simulink model "ieee80211n"  (Simulink 6.0)
settings: Solver=VariableStepDiscrete  StartTime=0.0  StopTime=inf  RelTol=1e-3
PreLoadFcn:
  | load IEEE80211n_init;
values from neighbouring files (symbols this model uses):
  params =     [IEEE80211n_init.mat]    (also in IEEE80211n_settings.m = p)
undefined symbols (not defined in the file or in its folder): magnitude
libraries: commblkintrlv2 x196, dspsigops x143, simulink x136, commdigbbndam2 x98, dspmtrx3 x96, dspsigattribs x69, dspstat3 x38, commutil2 x32, commsequence2 x26, commcnvcod2 x10, dspindex x9, dspmlti3 x8
(part 3 of 12)

== system ieee80211n/cyclic prefix1 ==
  in : Inport  Port=1  LatchInput=off
  Add Cyclic Prefix : Selector  InputType=Matrix  Elements=[49:64 1:64]  Rows=params.TXCyclicPrefixIndices  Columns=-1  InputPortWidth=64
  "Cyclic shift, SS2" : Subsystem
      mask Display: disp('Cyclic Shift\nDelay')
  out : Outport
  wires:
  Add Cyclic Prefix/1 -> out/1
  in/1 -> "Cyclic shift, SS2"/1(in)
  "Cyclic shift, SS2"/1(out) -> Add Cyclic Prefix/1

== system ieee80211n/cyclic prefix2 ==
  in : Inport  Port=1  LatchInput=off
  Add Cyclic Prefix : Selector  InputType=Matrix  Elements=[49:64 1:64]  Rows=params.TXCyclicPrefixIndices  Columns=-1  InputPortWidth=64
  "Cyclic shift, SS3" : Subsystem
      mask Display: disp('Cyclic Shift\nDelay')
  out : Outport
  wires:
  Add Cyclic Prefix/1 -> out/1
  in/1 -> "Cyclic shift, SS3"/1(in)
  "Cyclic shift, SS3"/1(out) -> Add Cyclic Prefix/1

== system ieee80211n/cyclic prefix3 ==
  in : Inport  Port=1  LatchInput=off
  Add Cyclic Prefix : Selector  InputType=Matrix  Elements=[49:64 1:64]  Rows=params.TXCyclicPrefixIndices  Columns=-1  InputPortWidth=64
  "Cyclic shift, SS4" : Subsystem
      mask Display: disp('Cyclic Shift\nDelay')
  out : Outport
  wires:
  Add Cyclic Prefix/1 -> out/1
  in/1 -> "Cyclic shift, SS4"/1(in)
  "Cyclic shift, SS4"/1(out) -> Add Cyclic Prefix/1

== system ieee80211n/remove cyclic prefix ==
  In1 : Inport  Port=1  LatchInput=off
  Remove cyclic prefix : Selector  InputType=Matrix  Elements=[17:80]  Rows=params.RXCyclicPrefixIndices  Columns=-1  InputPortWidth=80
  Out1 : Outport
  wires:
  In1/1 -> Remove cyclic prefix/1
  Remove cyclic prefix/1 -> Out1/1

== system ieee80211n/remove cyclic prefix1 ==
  In1 : Inport  Port=1  LatchInput=off
  Remove cyclic prefix : Selector  InputType=Matrix  Elements=[17:80]  Rows=params.RXCyclicPrefixIndices  Columns=-1  InputPortWidth=80
  Out1 : Outport
  wires:
  In1/1 -> Remove cyclic prefix/1
  Remove cyclic prefix/1 -> Out1/1

== system ieee80211n/remove cyclic prefix2 ==
  In1 : Inport  Port=1  LatchInput=off
  Remove cyclic prefix : Selector  InputType=Matrix  Elements=[17:80]  Rows=params.RXCyclicPrefixIndices  Columns=-1  InputPortWidth=80
  Out1 : Outport
  wires:
  In1/1 -> Remove cyclic prefix/1
  Remove cyclic prefix/1 -> Out1/1

== system ieee80211n/remove cyclic prefix3 ==
  In1 : Inport  Port=1  LatchInput=off
  Remove cyclic prefix : Selector  InputType=Matrix  Elements=[17:80]  Rows=params.RXCyclicPrefixIndices  Columns=-1  InputPortWidth=80
  Out1 : Outport
  wires:
  In1/1 -> Remove cyclic prefix/1
  Remove cyclic prefix/1 -> Out1/1

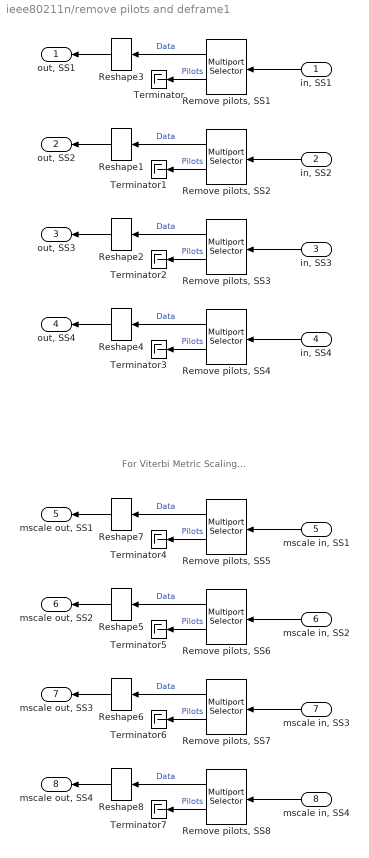
== system ieee80211n/remove pilots and deframe1 ==
  note: For Viterbi Metric Scaling...
  "in, SS1" : Inport  Orientation=left  Port=1  LatchInput=off
  "in, SS2" : Inport  Orientation=left  Port=2  LatchInput=off
  "in, SS3" : Inport  Orientation=left  Port=3  LatchInput=off
  "in, SS4" : Inport  Orientation=left  Port=4  LatchInput=off
  "mscale in, SS1" : Inport  Orientation=left  Port=5  LatchInput=off
  "mscale in, SS2" : Inport  Orientation=left  Port=6  LatchInput=off
  "mscale in, SS3" : Inport  Orientation=left  Port=7  LatchInput=off
  "mscale in, SS4" : Inport  Orientation=left  Port=8  LatchInput=off
  Remove pilots, SS{1..8} (8 alike) : dspindex/Multiport Selector  Orientation=left  rowsOrCols=Rows  idxCellArray="{[1:7 9:21 23:34 36:48 50:56], [8 22 35 49]}  % {[1:5 7:19 21:32 34:46 48:52], [6 20 33 47]}"  idxErrMode=Clip Index
  Reshape{1..8} (8 alike) : simulink/Math Operations/Reshape  Orientation=left  OutputDimensionality=Column vector  OutputDimensions=960
  Terminator{,1..7} (8 alike) : Terminator
  "out, SS1" : Outport  Orientation=left
  "out, SS2" : Outport  Orientation=left  Port=2
  "out, SS3" : Outport  Orientation=left  Port=3
  "out, SS4" : Outport  Orientation=left  Port=4
  "mscale out, SS1" : Outport  Orientation=left  Port=5
  "mscale out, SS2" : Outport  Orientation=left  Port=6
  "mscale out, SS3" : Outport  Orientation=left  Port=7
  "mscale out, SS4" : Outport  Orientation=left  Port=8
  wires:
  "Remove pilots, SS1"/2 -> Terminator/1  "Pilots"
  "Remove pilots, SS1"/1 -> Reshape3/1  "Data"
  Reshape3/1 -> "out, SS1"/1
  "in, SS1"/1 -> "Remove pilots, SS1"/1
  "Remove pilots, SS2"/2 -> Terminator1/1  "Pilots"
  "Remove pilots, SS2"/1 -> Reshape1/1  "Data"
  Reshape1/1 -> "out, SS2"/1
  "in, SS2"/1 -> "Remove pilots, SS2"/1
  "Remove pilots, SS3"/2 -> Terminator2/1  "Pilots"
  "Remove pilots, SS3"/1 -> Reshape2/1  "Data"
  Reshape2/1 -> "out, SS3"/1
  "in, SS3"/1 -> "Remove pilots, SS3"/1
  "Remove pilots, SS4"/2 -> Terminator3/1  "Pilots"
  "Remove pilots, SS4"/1 -> Reshape4/1  "Data"
  Reshape4/1 -> "out, SS4"/1
  "in, SS4"/1 -> "Remove pilots, SS4"/1
  "Remove pilots, SS5"/2 -> Terminator4/1  "Pilots"
  "Remove pilots, SS5"/1 -> Reshape7/1  "Data"
  Reshape7/1 -> "mscale out, SS1"/1
  "mscale in, SS1"/1 -> "Remove pilots, SS5"/1
  "Remove pilots, SS6"/2 -> Terminator5/1  "Pilots"
  "Remove pilots, SS6"/1 -> Reshape5/1  "Data"
  Reshape5/1 -> "mscale out, SS2"/1
  "mscale in, SS2"/1 -> "Remove pilots, SS6"/1
  "Remove pilots, SS7"/2 -> Terminator6/1  "Pilots"
  "Remove pilots, SS7"/1 -> Reshape6/1  "Data"
  Reshape6/1 -> "mscale out, SS3"/1
  "mscale in, SS3"/1 -> "Remove pilots, SS7"/1
  "Remove pilots, SS8"/2 -> Terminator7/1  "Pilots"
  "Remove pilots, SS8"/1 -> Reshape8/1  "Data"
  Reshape8/1 -> "mscale out, SS4"/1
  "mscale in, SS4"/1 -> "Remove pilots, SS8"/1

== system ieee80211n/remove pilots and training ==
  in : Inport  Port=1  LatchInput=off
  Frame Status Conversion1 : dspsigattribs/Frame Status Conversion  growRefPort=off  outframe=Sample-based
  Remove DC component : Selector  InputType=Matrix  Elements=[1:26 27:]  Rows=[1:26 28:53]  Columns=-1  InputPortWidth=53
  Remove training and pilots : Selector  InputType=Matrix  Elements=[17:80]  Rows=[1:5 7:19 21:32 34:46 48:52]  Columns=params.OFDMTrainPerFrame+1:params.OFDMTotSymPerFrame  InputPortWidth=80
  Reshape5 : simulink/Math Operations/Reshape  OutputDimensionality=Column vector  OutputDimensions=960
  out : Outport
  wires:
  Remove training and pilots/1 -> Reshape5/1
  Remove DC component/1 -> Remove training and pilots/1
  in/1 -> Remove DC component/1
  Reshape5/1 -> Frame Status Conversion1/1
  Frame Status Conversion1/1 -> out/1

== system ieee80211n/training ==
  Frame Status Conversion{1..4} (4 alike) : dspsigattribs/Frame Status Conversion  Orientation=left  growRefPort=off  outframe=Frame-based
  "Training, SS1" : Constant  Orientation=left  Value=params.HT20_long_training_seq_ss1
  "Training, SS2" : Constant  Orientation=left  Value=params.HT20_long_training_seq_ss2
  "Training, SS3" : Constant  Orientation=left  Value=params.HT20_long_training_seq_ss3
  "Training, SS4" : Constant  Orientation=left  Value=params.HT20_long_training_seq_ss4
  "Out, SS1" : Outport  Orientation=left
  "Out, SS2" : Outport  Orientation=left  Port=2
  "Out, SS3" : Outport  Orientation=left  Port=3
  "Out, SS4" : Outport  Orientation=left  Port=4
  wires:
  "Training, SS1"/1 -> Frame Status Conversion4/1
  Frame Status Conversion4/1 -> "Out, SS1"/1
  "Training, SS2"/1 -> Frame Status Conversion1/1
  Frame Status Conversion1/1 -> "Out, SS2"/1
  "Training, SS3"/1 -> Frame Status Conversion2/1
  Frame Status Conversion2/1 -> "Out, SS3"/1
  "Training, SS4"/1 -> Frame Status Conversion3/1
  Frame Status Conversion3/1 -> "Out, SS4"/1

== system ieee80211n/training sequence4 ==
  Combine Preamble, SS{1..4} (4 alike) : simulink/Math Operations/Matrix Concatenation  numInports=6  catMethod=Horizontal
  Modulator : Subsystem  mask(IEEE 802.11a modulator-coder bank.){nSymbolsPerFrame=params.OFDM_LSIG_SymPerFrame}
      mask prompts: nSymbolsPerFrame "Number of symbols per frame:"
      mask init:
      | if 0
      | numModulators = 8;
      | modulation = {'BPSK' 'BPSK' 'QPSK' 'QPSK' '16-QAM' '16-QAM' '64-QAM' '64-QAM'};
      | code = {'1/2' '3/4' '1/2' '3/4' '1/2' '3/4' '2/3' '3/4'};
      | 
      | % modulation-specific
      | TS1 = 'poly2trellis(7, [171 133])';
      | TS2 = 'poly2trellis(7, [133 171])';
      | trellisStructure = {TS1 TS1 TS1 TS1 TS1 TS1 TS2 TS2};
      | 
      | % code-specific
      | PV = {'[1]', '[1 1 1 0].''', '[1 1 1 0 0 1].''', '[1]'};
      | punctureVector = {PV{1} PV{3} PV{1} PV{3} PV{1} PV{3} PV{2} PV{3}};
      | 
      | for n = 1:numModulators
      |     blk = [gcb '/Modulator ' num2str(n)];
      |     set_param(blk, 'numSymbols', num2str(nSymbolsPerFrame));
      |     set_param(blk, 'modulation', modulation{n});
      |     set_param(blk, 'code', code{n});
      |     set_param(blk, 'trellisStructure', trellisStructure{n});
      |     set_param(blk, 'punctureVector', punctureVector{n});
      | end
      | end
      mask Display: disp('L-SIG')
  Modulator1 : Subsystem  mask(IEEE 802.11a modulator-coder bank.){nSymbolsPerFrame=params.OFDM_HTSIG_SymPerFrame}
      mask prompts: nSymbolsPerFrame "Number of symbols per frame:"
      mask init: same as ieee80211n/training sequence4/Modulator
      mask Display: disp('HT-SIG')
  Pilots : Subsystem
      mask Display: disp('Pilots')
  training sequence : Subsystem
      mask Display: disp('L-LTF')
  training sequence1 : Subsystem
      mask Display: disp('L-STF')
  training sequence2 : Subsystem
      mask Display: disp('HT-LTF')
  training sequence3 : Subsystem
      mask Display: disp('HT-STF')
  "out, SS1" : Outport
  "out, SS2" : Outport  Port=2
  "out, SS3" : Outport  Port=3
  "out, SS4" : Outport  Port=4
  wires:
  training sequence/1(out) -> "Combine Preamble, SS1"/2, "Combine Preamble, SS2"/2, "Combine Preamble, SS3"/2, "Combine Preamble, SS4"/2
  training sequence1/1(out) -> "Combine Preamble, SS1"/1, "Combine Preamble, SS2"/1, "Combine Preamble, SS3"/1, "Combine Preamble, SS4"/1
  training sequence2/1("out, SS1") -> "Combine Preamble, SS1"/6
  training sequence3/1("out, SS1") -> "Combine Preamble, SS1"/5
  "Combine Preamble, SS1"/1 -> "out, SS1"/1
  Modulator/1(out) -> "Combine Preamble, SS1"/3, "Combine Preamble, SS2"/3, "Combine Preamble, SS3"/3, "Combine Preamble, SS4"/3
  Modulator1/1(out) -> "Combine Preamble, SS1"/4, "Combine Preamble, SS2"/4, "Combine Preamble, SS3"/4, "Combine Preamble, SS4"/4
  Pilots/1(out) -> Modulator/1(pilot), Modulator1/1(pilot)
  "Combine Preamble, SS2"/1 -> "out, SS2"/1
  "Combine Preamble, SS3"/1 -> "out, SS3"/1
  "Combine Preamble, SS4"/1 -> "out, SS4"/1
  training sequence3/2("out, SS2") -> "Combine Preamble, SS2"/5
  training sequence3/3("out, SS3") -> "Combine Preamble, SS3"/5
  training sequence3/4("out, SS4") -> "Combine Preamble, SS4"/5
  training sequence2/2("out, SS2") -> "Combine Preamble, SS2"/6
  training sequence2/3("out, SS3") -> "Combine Preamble, SS3"/6
  training sequence2/4("out, SS4") -> "Combine Preamble, SS4"/6

== system ieee80211n/Adaptive  Modulation  Control/SNR up threshold ==
  idx : Inport  Port=1  LatchInput=off
  Constant : Constant
  Direct Look-Up Table (n-D) : simulink/Lookup Tables/Direct Lookup Table (n-D)  maskTabDims=1  explicitNumDims=1  outDims=Element  tabIsInput=off  mxTable=vector  clipFlag=Warning
  Sum : Sum  Inputs=|+-  SaturateOnIntegerOverflow=on
  val : Outport
  wires:
  idx/1 -> Sum/1
  Direct Look-Up Table (n-D)/1 -> val/1
  Sum/1 -> Direct Look-Up Table (n-D)/1
  Constant/1 -> Sum/2

== system ieee80211n/Data source/Binary source ==
  Enable : EnablePort
  Constant : Constant  Value=0.5
  Random Source : dspsrcs4/Random Source  SrcType=Uniform  NormMethod=Ziggurat  CltLength=12  Min=0  Max=1  Mean=0  Var=1  RepMode=Specify seed  rawSeed=61  Inherit=off  SampMode=Discrete  SampTime=sample_time  SampFrame=samp_per_frame  DataType=Double  OutComplex=Real
  Relational Operator : RelationalOperator  Operator=>  LogicOutDataTypeMode=Specify via dialog  LogicDataType=float('double')  InputSameDT=on
  data out : Outport  OutputWhenDisabled=reset  InitialOutput=0
  wires:
  Random Source/1 -> Relational Operator/1
  Constant/1 -> Relational Operator/2
  Relational Operator/1 -> data out/1

== system ieee80211n/Data source/Source enable ==
  mode : Inport  Port=1  LatchInput=off
  Constant : Constant  Value=(1:max(params.nS)).'
  Relational Operator1 : RelationalOperator  Operator=<=  LogicOutDataTypeMode=Specify via dialog  LogicDataType=float('double')  InputSameDT=on
  Unbuffer : dspbuff3/Unbuffer  ic=0
  slot size : IEEE80211a_lib/Select value  vector=params.nS.'
  enable : Outport
  wires:
  slot size/1 -> Relational Operator1/2
  Constant/1 -> Relational Operator1/1
  Relational Operator1/1 -> Unbuffer/1
  Unbuffer/1 -> enable/1
  mode/1 -> slot size/1

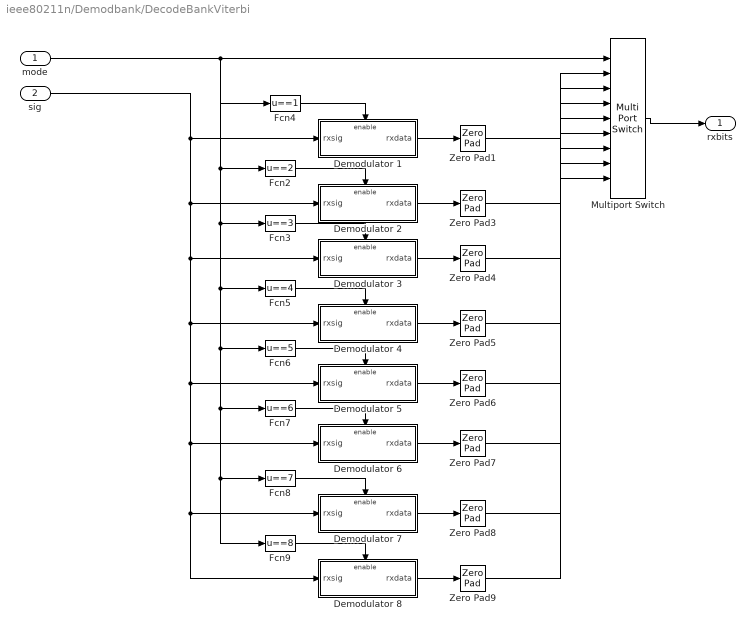
== system ieee80211n/Demodbank/DecodeBankViterbi ==
  mode : Inport  Port=1  LatchInput=off
  sig : Inport  Port=2  LatchInput=off
  Demodulator 1 : Subsystem  AncestorBlock=IEEE80211a_lib/Demodulator  TreatAsAtomicUnit=on  mask(Viterbi Decoder Bank.){numSymbols=1664, modulation=BPSK, code=1/2, trellisStructure=poly2trellis(7, [171 133]), punctureVector=[1], vtbd=128}
      mask prompts: numSymbols "Number of symbols per frame:"; trellisStructure "Trellis:"; punctureVector "Puncture vector:"; vtbd "Viterbi trace back depth:"
      mask help: Bank of different Viterbi decoders with same output frame size.
      mask init:
      | % number of bits per symbol
      | switch modulation
      | 	case 'BPSK', Nb1 = 1;
      | 	case 'QPSK', Nb1 = 2;
      | 	case '16-QAM', Nb1 = 4;
      | 	case '64-QAM', Nb1 = 6;
      | end
      | 
      | modOrder = 2.^Nb1;
      | Nb = numSymbols * Nb1; % tx bits per block
      | codeRate = str2num(strvcat(code)).';
      | bitsPerBlock = Nb .* codeRate;
      | s=max([Nb1/2 1]);
      | 
      | % interleaver
      | interleaverRows = 13;
      | if rem(Nb, interleaverRows)
      | 	error('Number of transmitted bits per block must be multiple of 16.')
      | end
      | interleaverCols = Nb / interleaverRows;
      | interleaverElements = [...
      |             s*floor( [0:Nb-1]/s ) + ...
      |             mod( ([0:Nb-1] + Nb - floor( interleaverRows*[0:Nb-1]/Nb ) ), s ) ...
      |             + 1]';
      mask Display:
      | disp(['Decoder\n' 'Rate=' code])
      | port_label('input', 1, ' ')
      | port_label('output', 1, ' ')
  Demodulator 2 : Subsystem  AncestorBlock=IEEE80211a_lib/Demodulator  TreatAsAtomicUnit=on  mask(Viterbi Decoder Bank.){numSymbols=1664, modulation=QPSK, code=1/2, trellisStructure=poly2trellis(7, [171 133]), punctureVector=[1], vtbd=128}
      mask prompts: numSymbols "Number of symbols per frame:"; trellisStructure "Trellis:"; punctureVector "Puncture vector:"; vtbd "Viterbi trace back depth:"
      mask help: Bank of different Viterbi decoders with same output frame size.
      mask init:
      | % number of bits per symbol
      | switch modulation
      | 	case 'BPSK', Nb1 = 1;
      | 	case 'QPSK', Nb1 = 2;
      | 	case '16-QAM', Nb1 = 4;
      | 	case '64-QAM', Nb1 = 6;
      | end
      | 
      | modOrder = 2.^Nb1;
      | Nb = numSymbols * Nb1; % tx bits per block
      | codeRate = str2num(strvcat(code)).';
      | bitsPerBlock = Nb .* codeRate;
      | s=max([Nb1/2 1]);
      | 
      | % interleaver
      | interleaverRows = 13;
      | if rem(Nb, interleaverRows)
      | 	error('Number of transmitted bits per block must be multiple of 16.')
      | end
      | interleaverCols = Nb / interleaverRows;
      | interleaverElements = [...
      |             s*floor( [0:Nb-1]/s ) + ...
      |             mod( ([0:Nb-1] + Nb - floor( interleaverRows*[0:Nb-1]/Nb ) ), s ) ...
      |             + 1]';
      mask Display:
      | disp(['Decoder\n' 'Rate=' code])
      | port_label('input', 1, ' ')
      | port_label('output', 1, ' ')
  Demodulator 3 : Subsystem  AncestorBlock=IEEE80211a_lib/Demodulator  TreatAsAtomicUnit=on  mask(Viterbi Decoder Bank.){numSymbols=1664, modulation=QPSK, code=3/4, trellisStructure=poly2trellis(7, [171 133]), punctureVector=[1 1 1 0 0 1].', vtbd=128}
      mask prompts: numSymbols "Number of symbols per frame:"; trellisStructure "Trellis:"; punctureVector "Puncture vector:"; vtbd "Viterbi trace back depth:"
      mask help: Bank of different Viterbi decoders with same output frame size.
      mask init: same as ieee80211n/Demodbank/DecodeBankViterbi/Demodulator 2
      mask Display:
      | disp(['Decoder\n' 'Rate=' code])
      | port_label('input', 1, ' ')
      | port_label('output', 1, ' ')
  Demodulator 4 : Subsystem  AncestorBlock=IEEE80211a_lib/Demodulator  TreatAsAtomicUnit=on  mask(Viterbi Decoder Bank.){numSymbols=1664, modulation=16-QAM, code=1/2, trellisStructure=poly2trellis(7, [171 133]), punctureVector=[1], vtbd=128}
      mask prompts: numSymbols "Number of symbols per frame:"; trellisStructure "Trellis:"; punctureVector "Puncture vector:"; vtbd "Viterbi trace back depth:"
      mask help: Bank of different Viterbi decoders with same output frame size.
      mask init: same as ieee80211n/Demodbank/DecodeBankViterbi/Demodulator 2
      mask Display:
      | disp(['Decoder\n' 'Rate=' code])
      | port_label('input', 1, ' ')
      | port_label('output', 1, ' ')
  Demodulator 5 : Subsystem  AncestorBlock=IEEE80211a_lib/Demodulator  TreatAsAtomicUnit=on  mask(Viterbi Decoder Bank.){numSymbols=1664, modulation=16-QAM, code=3/4, trellisStructure=poly2trellis(7, [171 133]), punctureVector=[1 1 1 0 0 1].', vtbd=128}
      mask prompts: numSymbols "Number of symbols per frame:"; trellisStructure "Trellis:"; punctureVector "Puncture vector:"; vtbd "Viterbi trace back depth:"
      mask help: Bank of different Viterbi decoders with same output frame size.
      mask init: same as ieee80211n/Demodbank/DecodeBankViterbi/Demodulator 2
      mask Display:
      | disp(['Decoder\n' 'Rate=' code])
      | port_label('input', 1, ' ')
      | port_label('output', 1, ' ')
  Demodulator 6 : Subsystem  AncestorBlock=IEEE80211a_lib/Demodulator  TreatAsAtomicUnit=on  mask(Viterbi Decoder Bank.){numSymbols=1664, modulation=64-QAM, code=2/3, trellisStructure=poly2trellis(7, [133 171]), punctureVector=[1 1 1 0].', vtbd=128}
      mask prompts: numSymbols "Number of symbols per frame:"; trellisStructure "Trellis:"; punctureVector "Puncture vector:"; vtbd "Viterbi trace back depth:"
      mask help: Bank of different Viterbi decoders with same output frame size.
      mask init: same as ieee80211n/Demodbank/DecodeBankViterbi/Demodulator 2
      mask Display:
      | disp(['Decoder\n' 'Rate=' code])
      | port_label('input', 1, ' ')
      | port_label('output', 1, ' ')
  Demodulator 7 : Subsystem  AncestorBlock=IEEE80211a_lib/Demodulator  TreatAsAtomicUnit=on  mask(Viterbi Decoder Bank.){numSymbols=1664, modulation=64-QAM, code=3/4, trellisStructure=poly2trellis(7, [133 171]), punctureVector=[1 1 1 0 0 1].', vtbd=128}
      mask prompts: numSymbols "Number of symbols per frame:"; trellisStructure "Trellis:"; punctureVector "Puncture vector:"; vtbd "Viterbi trace back depth:"
      mask help: Bank of different Viterbi decoders with same output frame size.
      mask init: same as ieee80211n/Demodbank/DecodeBankViterbi/Demodulator 2
      mask Display:
      | disp(['Decoder\n' 'Rate=' code])
      | port_label('input', 1, ' ')
      | port_label('output', 1, ' ')
  Demodulator 8 : Subsystem  AncestorBlock=IEEE80211a_lib/Demodulator  TreatAsAtomicUnit=on  mask(Viterbi Decoder Bank.){numSymbols=1664, modulation=64-QAM, code=5/6, trellisStructure=poly2trellis(7, [133 171]), punctureVector=[1 1 1 0 0 1 1 0 0 1].', vtbd=128}
      mask prompts: numSymbols "Number of symbols per frame:"; trellisStructure "Trellis:"; punctureVector "Puncture vector:"; vtbd "Viterbi trace back depth:"
      mask help: Bank of different Viterbi decoders with same output frame size.
      mask init: same as ieee80211n/Demodbank/DecodeBankViterbi/Demodulator 2
      mask Display:
      | disp(['Decoder\n' 'Rate=' code])
      | port_label('input', 1, ' ')
      | port_label('output', 1, ' ')
  Fcn2 : Fcn  Expr=u==2
  Fcn3 : Fcn  Expr=u==3
  Fcn4 : Fcn  Expr=u==1
  Fcn5 : Fcn  Expr=u==4
  Fcn6 : Fcn  Expr=u==5
  Fcn7 : Fcn  Expr=u==6
  Fcn8 : Fcn  Expr=u==7
  Fcn9 : Fcn  Expr=u==8
  Multiport Switch : MultiPortSwitch  Inputs=8  SaturateOnIntegerOverflow=on
  Zero Pad{1,3..9} (8 alike) : dspsigops/Zero Pad  padSigAt=End  zpadAlong=Columns  padNumOutRowsSpecMethod=User-specified  numOutRows=params.NSS*params.maxBitsPerBlock  padNumOutColsSpecMethod=User-specified  numOutCols=1  trunc_flag=None
      settings: AttributesFormatString=\n
  rxbits : Outport
  wires:
  sig/1 -> Demodulator 1/1(rxsig), Demodulator 3/1(rxsig), Demodulator 6/1(rxsig), Demodulator 7/1(rxsig), Demodulator 8/1(rxsig), Demodulator 5/1(rxsig), Demodulator 4/1(rxsig), Demodulator 2/1(rxsig)
  mode/1 -> Fcn4/1, Multiport Switch/1, Fcn7/1, Fcn8/1, Fcn9/1, Fcn6/1, Fcn5/1, Fcn3/1, Fcn2/1
  Multiport Switch/1 -> rxbits/1
  Zero Pad1/1 -> Multiport Switch/2
  Demodulator 7/1(rxdata) -> Zero Pad8/1
  Demodulator 6/1(rxdata) -> Zero Pad7/1
  Demodulator 5/1(rxdata) -> Zero Pad6/1
  Demodulator 3/1(rxdata) -> Zero Pad4/1
  Demodulator 4/1(rxdata) -> Zero Pad5/1
  Zero Pad3/1 -> Multiport Switch/3
  Zero Pad4/1 -> Multiport Switch/4
  Zero Pad5/1 -> Multiport Switch/5
  Zero Pad6/1 -> Multiport Switch/6
  Zero Pad7/1 -> Multiport Switch/7
  Zero Pad8/1 -> Multiport Switch/8
  Fcn4/1 -> Demodulator 1/Enable
  Fcn2/1 -> Demodulator 2/Enable
  Fcn3/1 -> Demodulator 3/Enable
  Fcn5/1 -> Demodulator 4/Enable
  Fcn6/1 -> Demodulator 5/Enable
  Fcn7/1 -> Demodulator 6/Enable
  Fcn8/1 -> Demodulator 7/Enable
  Demodulator 1/1(rxdata) -> Zero Pad1/1
  Demodulator 2/1(rxdata) -> Zero Pad3/1
  Demodulator 8/1(rxdata) -> Zero Pad9/1
  Zero Pad9/1 -> Multiport Switch/9
  Fcn9/1 -> Demodulator 8/Enable

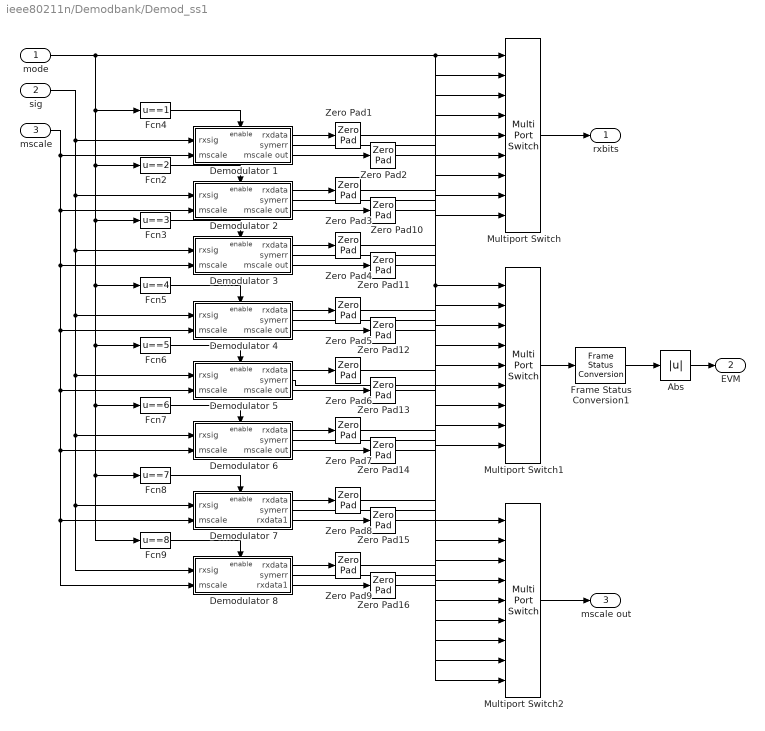
== system ieee80211n/Demodbank/Demod_ss1 ==
  mode : Inport  Port=1  LatchInput=off
  sig : Inport  Port=2  LatchInput=off
  mscale : Inport  Port=3  LatchInput=off
  Abs : Abs  SaturateOnIntegerOverflow=on
  Demodulator 1 : Subsystem  AncestorBlock=IEEE80211a_lib/Demodulator  TreatAsAtomicUnit=on  mask(QAM Demodulator-Decoder.){numSymbols=832, modulation=BPSK, code=1/2, trellisStructure=poly2trellis(7, [171 133]), punctureVector=[1], vtbd=128}
      mask prompts: numSymbols "Number of symbols per frame:"; trellisStructure "Trellis:"; punctureVector "Puncture vector:"; vtbd "Viterbi trace back depth:"
      mask help: Demodulator has option to zero-pad output, so that a bank of different modulators can share the same output frame size.
      mask init: same as ieee80211n/Demodbank/DecodeBankViterbi/Demodulator 1
      mask Display:
      | disp(['Demodulator\n' modulation ' ' code])
      | port_label('input', 1, ' ')
      | port_label('output', 1, ' ')
      | port_label('output', 2, 'err')
  Demodulator 2 : Subsystem  AncestorBlock=IEEE80211a_lib/Demodulator  TreatAsAtomicUnit=on  mask(QAM Demodulator-Decoder.){numSymbols=832, modulation=QPSK, code=1/2, trellisStructure=poly2trellis(7, [171 133]), punctureVector=[1], vtbd=128}
      mask prompts: numSymbols "Number of symbols per frame:"; trellisStructure "Trellis:"; punctureVector "Puncture vector:"; vtbd "Viterbi trace back depth:"
      mask help: Demodulator has option to zero-pad output, so that a bank of different modulators can share the same output frame size.
      mask init: same as ieee80211n/Demodbank/DecodeBankViterbi/Demodulator 2
      mask Display:
      | disp(['Demodulator\n' modulation ' ' code])
      | port_label('input', 1, ' ')
      | port_label('output', 1, ' ')
      | port_label('output', 2, 'err')
  Demodulator 3 : Subsystem  AncestorBlock=IEEE80211a_lib/Demodulator  TreatAsAtomicUnit=on  mask(QAM Demodulator-Decoder.){numSymbols=832, modulation=QPSK, code=3/4, trellisStructure=poly2trellis(7, [171 133]), punctureVector=[1 1 1 0 0 1].', vtbd=128}
      mask prompts: numSymbols "Number of symbols per frame:"; trellisStructure "Trellis:"; punctureVector "Puncture vector:"; vtbd "Viterbi trace back depth:"
      mask help: Demodulator has option to zero-pad output, so that a bank of different modulators can share the same output frame size.
      mask init: same as ieee80211n/Demodbank/DecodeBankViterbi/Demodulator 2
      mask Display:
      | disp(['Demodulator\n' modulation ' ' code])
      | port_label('input', 1, ' ')
      | port_label('output', 1, ' ')
      | port_label('output', 2, 'err')
  Demodulator 4 : Subsystem  AncestorBlock=IEEE80211a_lib/Demodulator  TreatAsAtomicUnit=on  mask(QAM Demodulator-Decoder.){numSymbols=832, modulation=16-QAM, code=1/2, trellisStructure=poly2trellis(7, [171 133]), punctureVector=[1], vtbd=128}
      mask prompts: numSymbols "Number of symbols per frame:"; trellisStructure "Trellis:"; punctureVector "Puncture vector:"; vtbd "Viterbi trace back depth:"
      mask help: Demodulator has option to zero-pad output, so that a bank of different modulators can share the same output frame size.
      mask init: same as ieee80211n/Demodbank/DecodeBankViterbi/Demodulator 2
      mask Display:
      | disp(['Demodulator\n' modulation ' ' code])
      | port_label('input', 1, ' ')
      | port_label('output', 1, ' ')
      | port_label('output', 2, 'err')
  Demodulator 5 : Subsystem  AncestorBlock=IEEE80211a_lib/Demodulator  TreatAsAtomicUnit=on  mask(QAM Demodulator-Decoder.){numSymbols=832, modulation=16-QAM, code=3/4, trellisStructure=poly2trellis(7, [171 133]), punctureVector=[1 1 1 0 0 1].', vtbd=128}
      mask prompts: numSymbols "Number of symbols per frame:"; trellisStructure "Trellis:"; punctureVector "Puncture vector:"; vtbd "Viterbi trace back depth:"
      mask help: Demodulator has option to zero-pad output, so that a bank of different modulators can share the same output frame size.
      mask init: same as ieee80211n/Demodbank/DecodeBankViterbi/Demodulator 2
      mask Display:
      | disp(['Demodulator\n' modulation ' ' code])
      | port_label('input', 1, ' ')
      | port_label('output', 1, ' ')
      | port_label('output', 2, 'err')
  Demodulator 6 : Subsystem  AncestorBlock=IEEE80211a_lib/Demodulator  TreatAsAtomicUnit=on  mask(QAM Demodulator-Decoder.){numSymbols=832, modulation=64-QAM, code=2/3, trellisStructure=poly2trellis(7, [133 171]), punctureVector=[1 1 1 0].', vtbd=128}
      mask prompts: numSymbols "Number of symbols per frame:"; trellisStructure "Trellis:"; punctureVector "Puncture vector:"; vtbd "Viterbi trace back depth:"
      mask help: Demodulator has option to zero-pad output, so that a bank of different modulators can share the same output frame size.
      mask init: same as ieee80211n/Demodbank/DecodeBankViterbi/Demodulator 2
      mask Display:
      | disp(['Demodulator\n' modulation ' ' code])
      | port_label('input', 1, ' ')
      | port_label('output', 1, ' ')
      | port_label('output', 2, 'err')
  Demodulator 7 : Subsystem  AncestorBlock=IEEE80211a_lib/Demodulator  TreatAsAtomicUnit=on  mask(QAM Demodulator-Decoder.){numSymbols=832, modulation=64-QAM, code=3/4, trellisStructure=poly2trellis(7, [133 171]), punctureVector=[1 1 1 0 0 1].', vtbd=12}
      mask prompts: numSymbols "Number of symbols per frame:"; trellisStructure "Trellis:"; punctureVector "Puncture vector:"; vtbd "Viterbi trace back depth:"
      mask help: Demodulator has option to zero-pad output, so that a bank of different modulators can share the same output frame size.
      mask init: same as ieee80211n/Demodbank/DecodeBankViterbi/Demodulator 2
      mask Display:
      | disp(['Demodulator\n' modulation ' ' code])
      | port_label('input', 1, ' ')
      | port_label('output', 1, ' ')
      | port_label('output', 2, 'err')
  Demodulator 8 : Subsystem  AncestorBlock=IEEE80211a_lib/Demodulator  TreatAsAtomicUnit=on  mask(QAM Demodulator-Decoder.){numSymbols=832, modulation=64-QAM, code=5/6, trellisStructure=poly2trellis(7, [133 171]), punctureVector=[1 1 1 0 0 1 1 0 0 1].', vtbd=128}
      mask prompts: numSymbols "Number of symbols per frame:"; trellisStructure "Trellis:"; punctureVector "Puncture vector:"; vtbd "Viterbi trace back depth:"
      mask help: Demodulator has option to zero-pad output, so that a bank of different modulators can share the same output frame size.
      mask init: same as ieee80211n/Demodbank/DecodeBankViterbi/Demodulator 2
      mask Display:
      | disp(['Demodulator\n' modulation ' ' code])
      | port_label('input', 1, ' ')
      | port_label('output', 1, ' ')
      | port_label('output', 2, 'err')
  Fcn2 : Fcn  Expr=u==2
  Fcn3 : Fcn  Expr=u==3
  Fcn4 : Fcn  Expr=u==1
  Fcn5 : Fcn  Expr=u==4
  Fcn6 : Fcn  Expr=u==5
  Fcn7 : Fcn  Expr=u==6
  Fcn8 : Fcn  Expr=u==7
  Fcn9 : Fcn  Expr=u==8
  Frame Status Conversion1 : dspsigattribs/Frame Status Conversion  growRefPort=off  outframe=Sample-based
  Multiport Switch : MultiPortSwitch  Inputs=8  SaturateOnIntegerOverflow=on
  Multiport Switch1 : MultiPortSwitch  Inputs=8  SaturateOnIntegerOverflow=on
  Multiport Switch2 : MultiPortSwitch  Inputs=8  SaturateOnIntegerOverflow=on
  Zero Pad{1..16} (16 alike) : dspsigops/Zero Pad  padSigAt=End  zpadAlong=Columns  padNumOutRowsSpecMethod=User-specified  numOutRows=params.maxTxBitsPerBlock  padNumOutColsSpecMethod=User-specified  numOutCols=1  trunc_flag=None
      settings: AttributesFormatString=\n
  rxbits : Outport
  EVM : Outport  Port=2
  mscale out : Outport  Port=3
  wires:
  sig/1 -> Demodulator 1/1(rxsig), Demodulator 3/1(rxsig), Demodulator 6/1(rxsig), Demodulator 7/1(rxsig), Demodulator 8/1(rxsig), Demodulator 5/1(rxsig), Demodulator 4/1(rxsig), Demodulator 2/1(rxsig)
  mode/1 -> Multiport Switch/1, Multiport Switch1/1, Multiport Switch2/1, Fcn4/1, Fcn7/1, Fcn8/1, Fcn9/1, Fcn6/1, Fcn5/1, Fcn3/1, Fcn2/1
  Multiport Switch/1 -> rxbits/1
  Zero Pad1/1 -> Multiport Switch/2
  Demodulator 7/1(rxdata) -> Zero Pad8/1
  Demodulator 6/1(rxdata) -> Zero Pad7/1
  Demodulator 5/1(rxdata) -> Zero Pad6/1
  Demodulator 3/1(rxdata) -> Zero Pad4/1
  Demodulator 4/1(rxdata) -> Zero Pad5/1
  Multiport Switch1/1 -> Frame Status Conversion1/1
  Demodulator 1/2(symerr) -> Multiport Switch1/2
  Demodulator 2/2(symerr) -> Multiport Switch1/3
  Demodulator 4/2(symerr) -> Multiport Switch1/5
  Demodulator 5/2(symerr) -> Multiport Switch1/6
  Demodulator 6/2(symerr) -> Multiport Switch1/7
  Demodulator 7/2(symerr) -> Multiport Switch1/8
  Demodulator 3/2(symerr) -> Multiport Switch1/4
  Zero Pad3/1 -> Multiport Switch/3
  Zero Pad4/1 -> Multiport Switch/4
  Zero Pad5/1 -> Multiport Switch/5
  Zero Pad6/1 -> Multiport Switch/6
  Zero Pad7/1 -> Multiport Switch/7
  Zero Pad8/1 -> Multiport Switch/8
  Fcn4/1 -> Demodulator 1/Enable
  Fcn2/1 -> Demodulator 2/Enable
  Fcn3/1 -> Demodulator 3/Enable
  Fcn5/1 -> Demodulator 4/Enable
  Fcn6/1 -> Demodulator 5/Enable
  Fcn7/1 -> Demodulator 6/Enable
  Fcn8/1 -> Demodulator 7/Enable
  Demodulator 1/1(rxdata) -> Zero Pad1/1
  Demodulator 2/1(rxdata) -> Zero Pad3/1
  Frame Status Conversion1/1 -> Abs/1
  Abs/1 -> EVM/1
  Demodulator 8/1(rxdata) -> Zero Pad9/1
  Demodulator 8/2(symerr) -> Multiport Switch1/9
  Zero Pad9/1 -> Multiport Switch/9
  Fcn9/1 -> Demodulator 8/Enable
  mscale/1 -> Demodulator 8/2(mscale), Demodulator 7/2(mscale), Demodulator 6/2(mscale), Demodulator 5/2(mscale), Demodulator 4/2(mscale), Demodulator 3/2(mscale), Demodulator 2/2(mscale), Demodulator 1/2(mscale)
  Multiport Switch2/1 -> mscale out/1
  Demodulator 1/3(mscale out) -> Zero Pad2/1
  Demodulator 2/3(mscale out) -> Zero Pad10/1
  Demodulator 3/3(mscale out) -> Zero Pad11/1
  Demodulator 4/3(mscale out) -> Zero Pad12/1
  Demodulator 5/3(mscale out) -> Zero Pad13/1
  Demodulator 6/3(mscale out) -> Zero Pad14/1
  Demodulator 7/3(rxdata1) -> Zero Pad15/1
  Demodulator 8/3(rxdata1) -> Zero Pad16/1
  Zero Pad2/1 -> Multiport Switch2/2
  Zero Pad10/1 -> Multiport Switch2/3
  Zero Pad11/1 -> Multiport Switch2/4
  Zero Pad12/1 -> Multiport Switch2/5
  Zero Pad13/1 -> Multiport Switch2/6
  Zero Pad14/1 -> Multiport Switch2/7
  Zero Pad15/1 -> Multiport Switch2/8
  Zero Pad16/1 -> Multiport Switch2/9

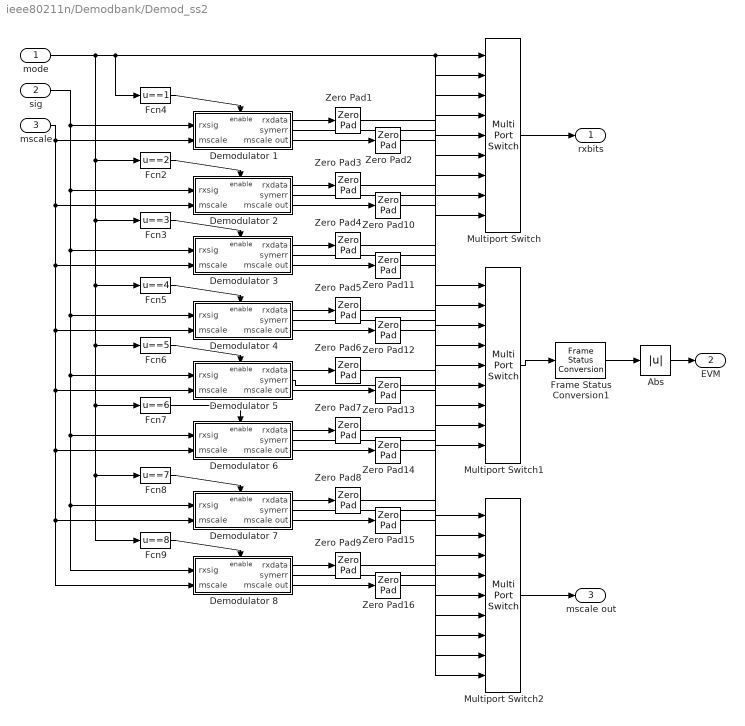
== system ieee80211n/Demodbank/Demod_ss2 ==
  mode : Inport  Port=1  LatchInput=off
  sig : Inport  Port=2  LatchInput=off
  mscale : Inport  Port=3  LatchInput=off
  Abs : Abs  SaturateOnIntegerOverflow=on
  Demodulator 1 : Subsystem  AncestorBlock=IEEE80211a_lib/Demodulator  TreatAsAtomicUnit=on  mask(QAM Demodulator-Decoder.){numSymbols=832, modulation=BPSK, code=1/2, trellisStructure=poly2trellis(7, [171 133]), punctureVector=[1], vtbd=128}
      mask prompts: numSymbols "Number of symbols per frame:"; trellisStructure "Trellis:"; punctureVector "Puncture vector:"; vtbd "Viterbi trace back depth:"
      mask help: Demodulator has option to zero-pad output, so that a bank of different modulators can share the same output frame size.
      mask init:
      | % number of bits per symbol
      | switch modulation
      | 	case 'BPSK', Nb1 = 1;
      | 	case 'QPSK', Nb1 = 2;
      | 	case '16-QAM', Nb1 = 4;
      | 	case '64-QAM', Nb1 = 6;
      | end
      | 
      | modOrder = 2.^Nb1;
      | Nb = numSymbols * Nb1; % tx bits per block
      | codeRate = str2num(strvcat(code)).';
      | bitsPerBlock = Nb .* codeRate;
      | s=max([Nb1/2 1]);
      | 
      | % interleaver
      | interleaverRows = 13;
      | if rem(Nb, interleaverRows)
      | 	error('Number of transmitted bits per block must be multiple of 16.')
      | end
      | interleaverCols = Nb / interleaverRows;
      | interleaverElements = [...
      |             s*floor( [0:Nb-1]/s ) + ...
      |             mod( ([0:Nb-1] + Nb - floor( interleaverRows*[0:Nb-1]/Nb ) ), s ) ...
      |             + 1]';
      | 	
      | if 1 %%%%%%%%%%%%%%%%%%%%%%%%
      | % freq rotation interleaver
      | iss = 1;
      | freqRotNum = 2*11;  % 20MHz channel
      | freqRotInterleaverElements = [...
      |             mod([0:Nb-1] - (mod(2*iss, 3) + 3*floor(iss/3)*freqRotNum*Nb1), Nb) ...
      |             + 1]';
      | end   %%%%%%%%%%%%%%%%%%%%%%%%
      mask Display:
      | disp(['Demodulator\n' modulation ' ' code])
      | port_label('input', 1, ' ')
      | port_label('output', 1, ' ')
      | port_label('output', 2, 'err')
  Demodulator 2 : Subsystem  AncestorBlock=IEEE80211a_lib/Demodulator  TreatAsAtomicUnit=on  mask(QAM Demodulator-Decoder.){numSymbols=832, modulation=QPSK, code=1/2, trellisStructure=poly2trellis(7, [171 133]), punctureVector=[1], vtbd=128}
      mask prompts: numSymbols "Number of symbols per frame:"; trellisStructure "Trellis:"; punctureVector "Puncture vector:"; vtbd "Viterbi trace back depth:"
      mask help: Demodulator has option to zero-pad output, so that a bank of different modulators can share the same output frame size.
      mask init: same as ieee80211n/Demodbank/Demod_ss2/Demodulator 1
      mask Display:
      | disp(['Demodulator\n' modulation ' ' code])
      | port_label('input', 1, ' ')
      | port_label('output', 1, ' ')
      | port_label('output', 2, 'err')
  Demodulator 3 : Subsystem  AncestorBlock=IEEE80211a_lib/Demodulator  TreatAsAtomicUnit=on  mask(QAM Demodulator-Decoder.){numSymbols=832, modulation=QPSK, code=3/4, trellisStructure=poly2trellis(7, [171 133]), punctureVector=[1 1 1 0 0 1].', vtbd=128}
      mask prompts: numSymbols "Number of symbols per frame:"; trellisStructure "Trellis:"; punctureVector "Puncture vector:"; vtbd "Viterbi trace back depth:"
      mask help: Demodulator has option to zero-pad output, so that a bank of different modulators can share the same output frame size.
      mask init: same as ieee80211n/Demodbank/Demod_ss2/Demodulator 1
      mask Display:
      | disp(['Demodulator\n' modulation ' ' code])
      | port_label('input', 1, ' ')
      | port_label('output', 1, ' ')
      | port_label('output', 2, 'err')
  Demodulator 4 : Subsystem  AncestorBlock=IEEE80211a_lib/Demodulator  TreatAsAtomicUnit=on  mask(QAM Demodulator-Decoder.){numSymbols=832, modulation=16-QAM, code=1/2, trellisStructure=poly2trellis(7, [171 133]), punctureVector=[1], vtbd=128}
      mask prompts: numSymbols "Number of symbols per frame:"; trellisStructure "Trellis:"; punctureVector "Puncture vector:"; vtbd "Viterbi trace back depth:"
      mask help: Demodulator has option to zero-pad output, so that a bank of different modulators can share the same output frame size.
      mask init: same as ieee80211n/Demodbank/Demod_ss2/Demodulator 1
      mask Display:
      | disp(['Demodulator\n' modulation ' ' code])
      | port_label('input', 1, ' ')
      | port_label('output', 1, ' ')
      | port_label('output', 2, 'err')
  Demodulator 5 : Subsystem  AncestorBlock=IEEE80211a_lib/Demodulator  TreatAsAtomicUnit=on  mask(QAM Demodulator-Decoder.){numSymbols=832, modulation=16-QAM, code=3/4, trellisStructure=poly2trellis(7, [171 133]), punctureVector=[1 1 1 0 0 1].', vtbd=128}
      mask prompts: numSymbols "Number of symbols per frame:"; trellisStructure "Trellis:"; punctureVector "Puncture vector:"; vtbd "Viterbi trace back depth:"
      mask help: Demodulator has option to zero-pad output, so that a bank of different modulators can share the same output frame size.
      mask init: same as ieee80211n/Demodbank/Demod_ss2/Demodulator 1
      mask Display:
      | disp(['Demodulator\n' modulation ' ' code])
      | port_label('input', 1, ' ')
      | port_label('output', 1, ' ')
      | port_label('output', 2, 'err')
  Demodulator 6 : Subsystem  AncestorBlock=IEEE80211a_lib/Demodulator  TreatAsAtomicUnit=on  mask(QAM Demodulator-Decoder.){numSymbols=832, modulation=64-QAM, code=2/3, trellisStructure=poly2trellis(7, [133 171]), punctureVector=[1 1 1 0].', vtbd=128}
      mask prompts: numSymbols "Number of symbols per frame:"; trellisStructure "Trellis:"; punctureVector "Puncture vector:"; vtbd "Viterbi trace back depth:"
      mask help: Demodulator has option to zero-pad output, so that a bank of different modulators can share the same output frame size.
      mask init: same as ieee80211n/Demodbank/Demod_ss2/Demodulator 1
      mask Display:
      | disp(['Demodulator\n' modulation ' ' code])
      | port_label('input', 1, ' ')
      | port_label('output', 1, ' ')
      | port_label('output', 2, 'err')
  Demodulator 7 : Subsystem  AncestorBlock=IEEE80211a_lib/Demodulator  TreatAsAtomicUnit=on  mask(QAM Demodulator-Decoder.){numSymbols=832, modulation=64-QAM, code=3/4, trellisStructure=poly2trellis(7, [133 171]), punctureVector=[1 1 1 0 0 1].', vtbd=128}
      mask prompts: numSymbols "Number of symbols per frame:"; trellisStructure "Trellis:"; punctureVector "Puncture vector:"; vtbd "Viterbi trace back depth:"
      mask help: Demodulator has option to zero-pad output, so that a bank of different modulators can share the same output frame size.
      mask init: same as ieee80211n/Demodbank/Demod_ss2/Demodulator 1
      mask Display:
      | disp(['Demodulator\n' modulation ' ' code])
      | port_label('input', 1, ' ')
      | port_label('output', 1, ' ')
      | port_label('output', 2, 'err')
  Demodulator 8 : Subsystem  AncestorBlock=IEEE80211a_lib/Demodulator  TreatAsAtomicUnit=on  mask(QAM Demodulator-Decoder.){numSymbols=832, modulation=64-QAM, code=5/6, trellisStructure=poly2trellis(7, [133 171]), punctureVector=[1 1 1 0 0 1 1 0 0 1].', vtbd=128}
      mask prompts: numSymbols "Number of symbols per frame:"; trellisStructure "Trellis:"; punctureVector "Puncture vector:"; vtbd "Viterbi trace back depth:"
      mask help: Demodulator has option to zero-pad output, so that a bank of different modulators can share the same output frame size.
      mask init: same as ieee80211n/Demodbank/Demod_ss2/Demodulator 1
      mask Display:
      | disp(['Demodulator\n' modulation ' ' code])
      | port_label('input', 1, ' ')
      | port_label('output', 1, ' ')
      | port_label('output', 2, 'err')
  Fcn2 : Fcn  Expr=u==2
  Fcn3 : Fcn  Expr=u==3
  Fcn4 : Fcn  Expr=u==1
  Fcn5 : Fcn  Expr=u==4
  Fcn6 : Fcn  Expr=u==5
  Fcn7 : Fcn  Expr=u==6
  Fcn8 : Fcn  Expr=u==7
  Fcn9 : Fcn  Expr=u==8
  Frame Status Conversion1 : dspsigattribs/Frame Status Conversion  growRefPort=off  outframe=Sample-based
  Multiport Switch : MultiPortSwitch  Inputs=8  SaturateOnIntegerOverflow=on
  Multiport Switch1 : MultiPortSwitch  Inputs=8  SaturateOnIntegerOverflow=on
  Multiport Switch2 : MultiPortSwitch  Inputs=8  SaturateOnIntegerOverflow=on
  Zero Pad{1..16} (16 alike) : dspsigops/Zero Pad  padSigAt=End  zpadAlong=Columns  padNumOutRowsSpecMethod=User-specified  numOutRows=params.maxTxBitsPerBlock  padNumOutColsSpecMethod=User-specified  numOutCols=1  trunc_flag=None
      settings: AttributesFormatString=\n
  rxbits : Outport
  EVM : Outport  Port=2
  mscale out : Outport  Port=3
  wires:
  sig/1 -> Demodulator 1/1(rxsig), Demodulator 3/1(rxsig), Demodulator 6/1(rxsig), Demodulator 7/1(rxsig), Demodulator 8/1(rxsig), Demodulator 5/1(rxsig), Demodulator 4/1(rxsig), Demodulator 2/1(rxsig)
  mode/1 -> Multiport Switch1/1, Multiport Switch/1, Multiport Switch2/1, Fcn4/1, Fcn7/1, Fcn8/1, Fcn9/1, Fcn6/1, Fcn5/1, Fcn3/1, Fcn2/1
  Multiport Switch/1 -> rxbits/1
  Zero Pad1/1 -> Multiport Switch/2
  Demodulator 7/1(rxdata) -> Zero Pad8/1
  Demodulator 6/1(rxdata) -> Zero Pad7/1
  Demodulator 5/1(rxdata) -> Zero Pad6/1
  Demodulator 3/1(rxdata) -> Zero Pad4/1
  Demodulator 4/1(rxdata) -> Zero Pad5/1
  Multiport Switch1/1 -> Frame Status Conversion1/1
  Demodulator 1/2(symerr) -> Multiport Switch1/2
  Demodulator 2/2(symerr) -> Multiport Switch1/3
  Demodulator 4/2(symerr) -> Multiport Switch1/5
  Demodulator 5/2(symerr) -> Multiport Switch1/6
  Demodulator 6/2(symerr) -> Multiport Switch1/7
  Demodulator 7/2(symerr) -> Multiport Switch1/8
  Demodulator 3/2(symerr) -> Multiport Switch1/4
  Zero Pad3/1 -> Multiport Switch/3
  Zero Pad4/1 -> Multiport Switch/4
  Zero Pad5/1 -> Multiport Switch/5
  Zero Pad6/1 -> Multiport Switch/6
  Zero Pad7/1 -> Multiport Switch/7
  Zero Pad8/1 -> Multiport Switch/8
  Fcn4/1 -> Demodulator 1/Enable
  Fcn2/1 -> Demodulator 2/Enable
  Fcn3/1 -> Demodulator 3/Enable
  Fcn5/1 -> Demodulator 4/Enable
  Fcn6/1 -> Demodulator 5/Enable
  Fcn7/1 -> Demodulator 6/Enable
  Fcn8/1 -> Demodulator 7/Enable
  Demodulator 1/1(rxdata) -> Zero Pad1/1
  Demodulator 2/1(rxdata) -> Zero Pad3/1
  Frame Status Conversion1/1 -> Abs/1
  Abs/1 -> EVM/1
  Demodulator 8/1(rxdata) -> Zero Pad9/1
  Demodulator 8/2(symerr) -> Multiport Switch1/9
  Zero Pad9/1 -> Multiport Switch/9
  Fcn9/1 -> Demodulator 8/Enable
  Multiport Switch2/1 -> mscale out/1
  Demodulator 1/3(mscale out) -> Zero Pad2/1
  Demodulator 2/3(mscale out) -> Zero Pad10/1
  Demodulator 3/3(mscale out) -> Zero Pad11/1
  Demodulator 4/3(mscale out) -> Zero Pad12/1
  Demodulator 5/3(mscale out) -> Zero Pad13/1
  Demodulator 6/3(mscale out) -> Zero Pad14/1
  Demodulator 7/3(mscale out) -> Zero Pad15/1
  Demodulator 8/3(mscale out) -> Zero Pad16/1
  mscale/1 -> Demodulator 1/2(mscale), Demodulator 2/2(mscale), Demodulator 3/2(mscale), Demodulator 4/2(mscale), Demodulator 5/2(mscale), Demodulator 6/2(mscale), Demodulator 7/2(mscale), Demodulator 8/2(mscale)
  Zero Pad2/1 -> Multiport Switch2/2
  Zero Pad10/1 -> Multiport Switch2/3
  Zero Pad11/1 -> Multiport Switch2/4
  Zero Pad12/1 -> Multiport Switch2/5
  Zero Pad13/1 -> Multiport Switch2/6
  Zero Pad14/1 -> Multiport Switch2/7
  Zero Pad15/1 -> Multiport Switch2/8
  Zero Pad16/1 -> Multiport Switch2/9
